simulink model "zhengtiKalman"  (R2016a)
settings: Solver=VariableStepAuto  StartTime=0.0  StopTime=100  RelTol=1e-3
libraries: simulink x2
settings Model: Creator=24535  LastModifiedBy=24535

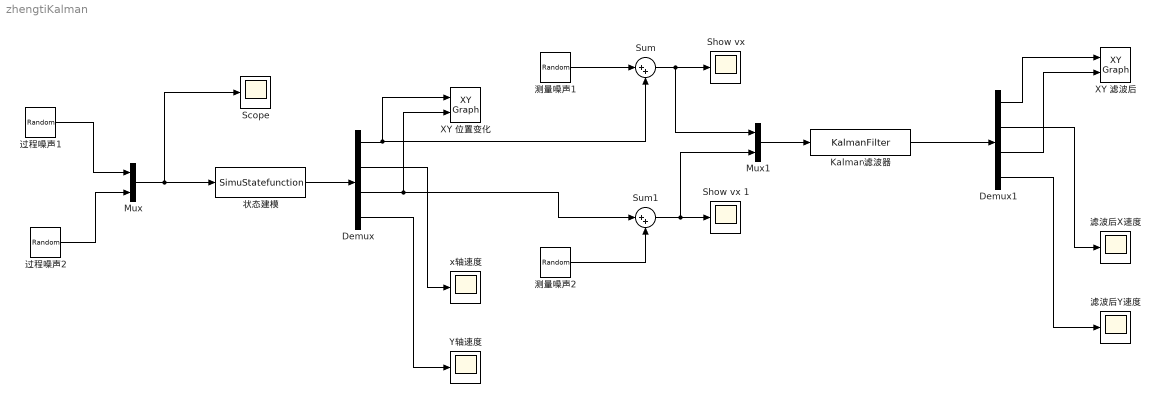
== system zhengtiKalman ==
  " 滤波后X速度" : Scope
  " 滤波后Y速度" : Scope
  " Show vx " : Scope
  " Show vx 1" : Scope
  " Y轴速度" : Scope
  " x轴速度" : Scope
  Demux : Demux
  Demux1 : Demux
  Kalman滤波器 : S-Function  FunctionName=KalmanFilter  SFunctionDeploymentMode=off  EnableBusSupport=off
  Mux : Mux  Inputs=2
  Mux1 : Mux  Inputs=2
  Scope : Scope
  Sum : Sum  Inputs=|++
  Sum1 : Sum  Inputs=|++
  XY 位置变化 : simulink/Sinks/XY Graph  xmin=0  xmax=600  ymin=0  ymax=600  st=-1
  XY 滤波后 : simulink/Sinks/XY Graph  xmin=0  xmax=600  ymin=0  ymax=600  st=-1
  测量噪声1 : RandomNumber  Variance=0.04  SampleTime=1
  测量噪声2 : RandomNumber  Variance=0.04  Seed=3  SampleTime=1
  状态建模 : S-Function  FunctionName=SimuStatefunction  SFunctionDeploymentMode=off  EnableBusSupport=off
  过程噪声1 : RandomNumber  Variance=0.0001  SampleTime=1
  过程噪声2 : RandomNumber  Variance=0.0009  Seed=3  SampleTime=1
  wires:
  过程噪声1/1 -> Mux/1
  过程噪声2/1 -> Mux/2
  Mux/1 -> Scope/1, 状态建模/1
  状态建模/1 -> Demux/1
  Demux/3 -> Sum1/1, XY 位置变化/2
  Demux/1 -> Sum/2, XY 位置变化/1
  Sum/1 -> Mux1/1, " Show vx "/1
  测量噪声1/1 -> Sum/1
  测量噪声2/1 -> Sum1/2
  Sum1/1 -> Mux1/2, " Show vx 1"/1
  Demux/2 -> " x轴速度"/1
  Demux/4 -> " Y轴速度"/1
  Mux1/1 -> Kalman滤波器/1
  Kalman滤波器/1 -> Demux1/1
  Demux1/3 -> XY 滤波后/2
  Demux1/1 -> XY 滤波后/1
  Demux1/2 -> " 滤波后X速度"/1
  Demux1/4 -> " 滤波后Y速度"/1
